simulink model "evse_twin"  (R2023b)
settings: Solver=VariableStepAuto  StartTime=0.0  StopTime=5  RelTol=1e-3
settings Model: Creator=dawid  LastModifiedBy=dawid
settings OptimizationCC: BooleanDataType=off

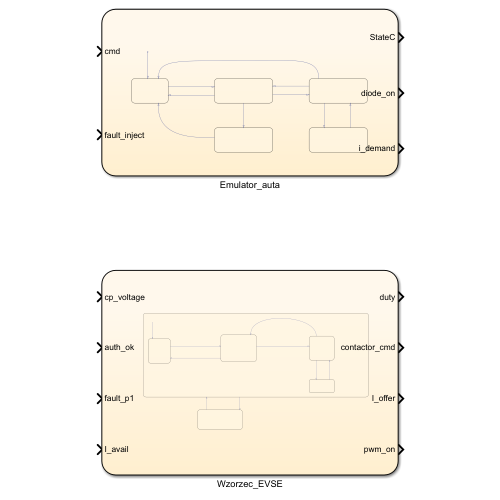
[thumbnail: Simulink's stored preview of the top-level diagram]
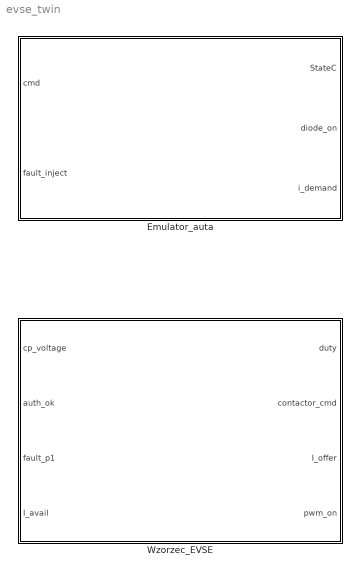
== system evse_twin ==
  Emulator_auta : Stateflow chart  TreatAsAtomicUnit=on
  Wzorzec_EVSE : Stateflow chart  TreatAsAtomicUnit=on

== stateflow chart evse_twin/Wzorzec_EVSE ==
  note: Petla 3 (aplikacja): auth_ok, I_avail = nastawy/limity (RFID, DLB, harmonogram).
  state Operating
    state Detected
      entry: pwm_on=1; I_offer=I_avail;
      duty=I_offer/0.6;
      contactor_cmd=0;
    state Charging
      entry: contactor_cmd=1;
      during: I_offer=I_avail;
      duty=I_offer/0.6;
    state Idle
      entry: pwm_on=0;
      duty=0;
      contactor_cmd=0;
      I_offer=0;
    state Ventilation
      entry: contactor_cmd=1;
    Charging -> Detected [order 1] : [cp_voltage>7.5 && cp_voltage<10.5]
    (default) -> Idle
    Idle -> Detected : [cp_voltage>7.5 && cp_voltage<10.5]
    Detected -> Charging [order 1] : [cp_voltage>4.5 && cp_voltage<7.5 && auth_ok==1]
    Detected -> Idle [order 2] : [cp_voltage>10.5]
    Charging -> Ventilation [order 2] : [cp_voltage>1.5 && cp_voltage<4.5]
    Ventilation -> Charging : [cp_voltage>4.5 && cp_voltage<7.5]
  state Tripped
    entry: contactor_cmd=0; pwm_on=0; duty=0;
  note: Petla 1 (bezpieczenstwo): fault_p1 = OR(RCD, PE, zwarcie CP, sklejenie). Weto nadrzedne.
  note: I_offer/duty: duty=I_offer/0.6 (10-85%). DLB: during w Charging sledzi I_avail.
  Tripped -> Operating : [fault_p1==0]
  Operating -> Tripped : [fault_p1==1]
  data: cp_voltage input; auth_ok input; fault_p1 input; I_avail input; duty output; contactor_cmd output; I_offer output; pwm_on output

== stateflow chart evse_twin/Emulator_auta ==
  note: Emulator auta: pasywny elektrycznie - wybiera rezystory/diode.
  state A_Unplugged
    entry: diode_on=0;
    StateC=0;
    i_demand=0;
  state B_Connected
    entry: diode_on=1;
    StateC=0;
    i_demand=0;
  state C_Ready
    entry: StateC=1;
    i_demand=16;
  state Fault
    entry: diode_on=0;
    StateC=0;
    i_demand=0;
  state D_Ventilation
    entry: StateC=1;
    i_demand=10;
  (default) -> A_Unplugged
  C_Ready -> A_Unplugged [order 3] : [cmd==0]
  C_Ready -> B_Connected [order 1] : [cmd==3]
  A_Unplugged -> B_Connected : [cmd==1]
  B_Connected -> C_Ready [order 1] : [cmd==2]
  B_Connected -> A_Unplugged [order 2] : [cmd==0]
  Fault -> A_Unplugged : [fault_inject==0]
  B_Connected -> Fault [order 3] : [fault_inject==1]
  C_Ready -> D_Ventilation [order 2] : [cmd==4]
  D_Ventilation -> C_Ready : [cmd==2]
  data: cmd input; fault_inject input; StateC output; diode_on output; i_demand output
